simulink model "Simulink_lab2"  (R2023a)
settings: Solver=FixedStepAuto  StartTime=0.0  StopTime=10.0  FixedStep=1e-3  RelTol=1e-3
settings Model: Creator=mazen  LastModifiedBy=mazen

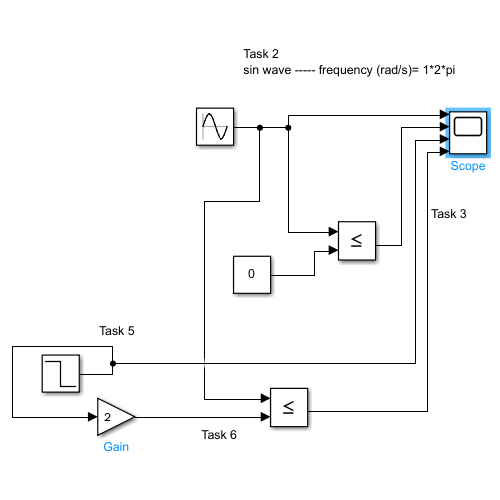
[thumbnail: Simulink's stored preview of the top-level diagram]
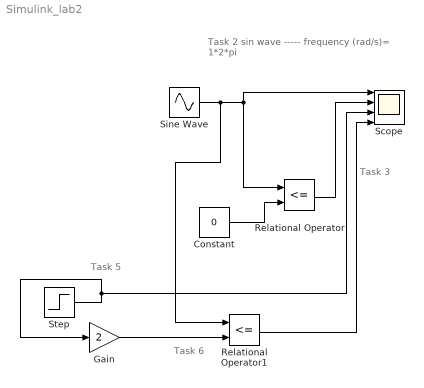
== system Simulink_lab2 ==
  note: Task 6
  note: Task 5
  note: Task 3
  note: Task 2
      | sin wave ----- frequency (rad/s)= 1*2*pi
  Constant : Constant  Value=0
  Gain : Gain  Gain=2
  Relational Operator : RelationalOperator  Operator=<=  OutDataTypeStr=boolean  RndMeth=Simplest  InputSameDT=off
  Relational Operator1 : RelationalOperator  Operator=<=  OutDataTypeStr=boolean  RndMeth=Simplest  InputSameDT=off
  Scope : Scope  NumInputPorts=4
  Sine Wave : Sin  Frequency=1*2*pi  SampleTime=0
  Step : Step  Before=2  SampleTime=0
  wires:
  Sine Wave/1 -> Relational Operator1/1, Relational Operator/1, Scope/1
  Constant/1 -> Relational Operator/2
  Relational Operator/1 -> Scope/2
  Step/1 -> Gain/1, Scope/3
  Gain/1 -> Relational Operator1/2
  Relational Operator1/1 -> Scope/4
